simulink model "DriveTrain"  (R2019b)
settings: Solver=VariableStepAuto  StartTime=0.0  StopTime=30  RelTol=1e-3
settings Model: Creator=jorge  LastModifiedBy=jorge

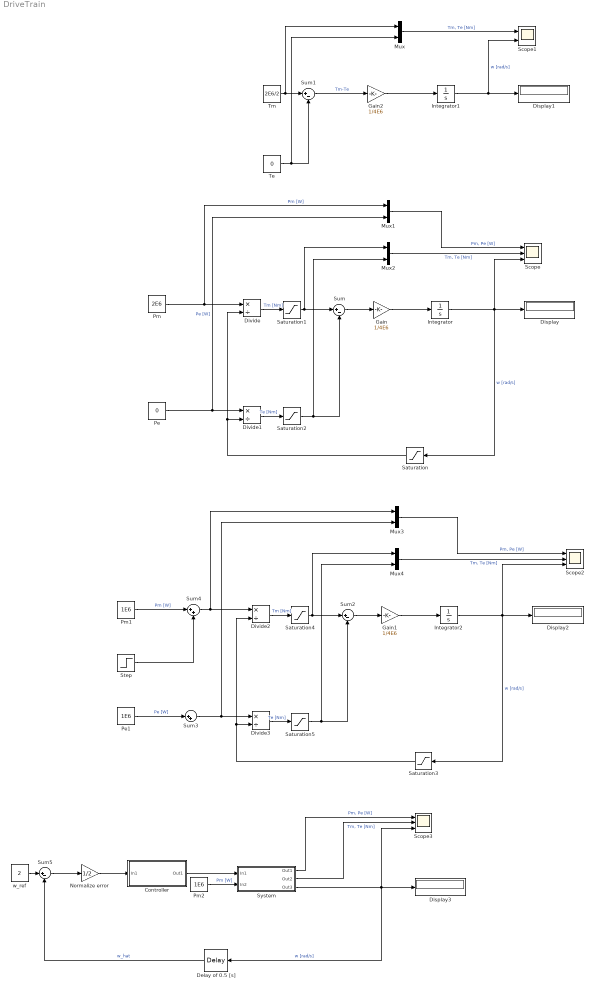
== system DriveTrain ==
  Controller : Subsystem
  Delay of 0.5 [s] : TransportDelay  DelayTime=0.5
  Display{,1..3} (4 alike) : Display
  Divide{,1..3} (4 alike) : Product  Inputs=*/
  Gain : Gain  Gain=1/4E6
  Gain1 : Gain  Gain=1/4E6
  Gain2 : Gain  Gain=1/4E6
  Integrator : Integrator
  Integrator1 : Integrator
  Integrator2 : Integrator  InitialCondition=2
  Mux{,1..4} (5 alike) : Mux  Inputs=2
  Normalize error : Gain  Gain=1/2
  Pe : Constant  Value=0
  Pe1 : Constant  Value=1E6
  Pm : Constant  Value=2E6
  Pm1 : Constant  Value=1E6
  Pm2 : Constant  Value=1E6
  Saturation : Saturate  UpperLimit=inf  LowerLimit=0.001
  Saturation1 : Saturate  UpperLimit=2E6
  Saturation2 : Saturate  UpperLimit=2E6  LowerLimit=0
  Saturation3 : Saturate  UpperLimit=inf  LowerLimit=0.001
  Saturation4 : Saturate  UpperLimit=2E6
  Saturation5 : Saturate  UpperLimit=2E6  LowerLimit=0
  Scope : Scope  NumInputPorts=3
  Scope1 : Scope  NumInputPorts=2
  Scope2 : Scope  NumInputPorts=3
  Scope3 : Scope  NumInputPorts=3
  Step : Step  After=2E5  SampleTime=0
  Sum{,1..2,5} (4 alike) : Sum  Inputs=|+-
  Sum3 : Sum  Inputs=|++
  Sum4 : Sum  Inputs=|++
  System : Subsystem
  Te : Constant  Value=0
  Tm : Constant  Value=2E6/2
  w_ref : Constant  Value=2
  wires:
  Integrator/1 -> Scope/3, Saturation/1, Display/1  "w [rad/s]"
  Gain/1 -> Integrator/1
  Gain2/1 -> Integrator1/1
  Sum1/1 -> Gain2/1  "Tm-Te"
  Integrator1/1 -> Scope1/2, Display1/1  "w [rad/s]"
  Te/1 -> Mux/2, Sum1/2
  Tm/1 -> Mux/1, Sum1/1
  Pm/1 -> Mux1/1, Divide/1  "Pm [W]"
  Saturation/1 -> Divide1/2, Divide/2
  Mux/1 -> Scope1/1  "Tm, Te [Nm]"
  Pe/1 -> Mux1/2, Divide1/1  "Pe [W]"
  Mux1/1 -> Scope/1  "Pm, Pe [W]"
  Sum/1 -> Gain/1
  Mux2/1 -> Scope/2  "Tm, Te [Nm]"
  Saturation1/1 -> Mux2/1, Sum/1
  Divide/1 -> Saturation1/1  "Tm [Nm]"
  Divide1/1 -> Saturation2/1  "Te [Nm]"
  Saturation2/1 -> Mux2/2, Sum/2
  Saturation4/1 -> Mux4/1, Sum2/1
  Divide3/1 -> Saturation5/1  "Te [Nm]"
  Gain1/1 -> Integrator2/1
  Integrator2/1 -> Scope2/3, Saturation3/1, Display2/1  "w [rad/s]"
  Divide2/1 -> Saturation4/1  "Tm [Nm]"
  Mux4/1 -> Scope2/2  "Tm, Te [Nm]"
  Mux3/1 -> Scope2/1  "Pm, Pe [W]"
  Saturation5/1 -> Mux4/2, Sum2/2
  Sum2/1 -> Gain1/1
  Saturation3/1 -> Divide3/2, Divide2/2
  Sum3/1 -> Mux3/2, Divide3/1
  Pe1/1 -> Sum3/1  "Pe [W]"
  Sum4/1 -> Mux3/1, Divide2/1
  Pm1/1 -> Sum4/1  "Pm [W]"
  Step/1 -> Sum4/2
  Pm2/1 -> System/2(In2)  "Pm [W]"
  Controller/1(Out1) -> System/1(In1)
  w_ref/1 -> Sum5/1
  Delay of 0.5 [s]/1 -> Sum5/2  "w_hat"
  System/1(Out1) -> Scope3/1  "Pm, Pe [W]"
  System/2(Out2) -> Scope3/2  "Tm, Te [Nm]"
  System/3(Out3) -> Scope3/3, Delay of 0.5 [s]/1, Display3/1  "w [rad/s]"
  Sum5/1 -> Normalize error/1
  Normalize error/1 -> Controller/1(In1)

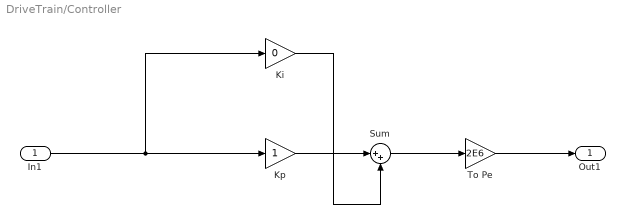
== system DriveTrain/Controller ==
  In1 : Inport
  Ki : Gain  Gain=0
  Kp : Gain
  Sum : Sum  Inputs=|++
  To Pe : Gain  Gain=2E6
  Out1 : Outport
  wires:
  In1/1 -> Ki/1, Kp/1
  Ki/1 -> Sum/2
  Kp/1 -> Sum/1
  Sum/1 -> To Pe/1
  To Pe/1 -> Out1/1

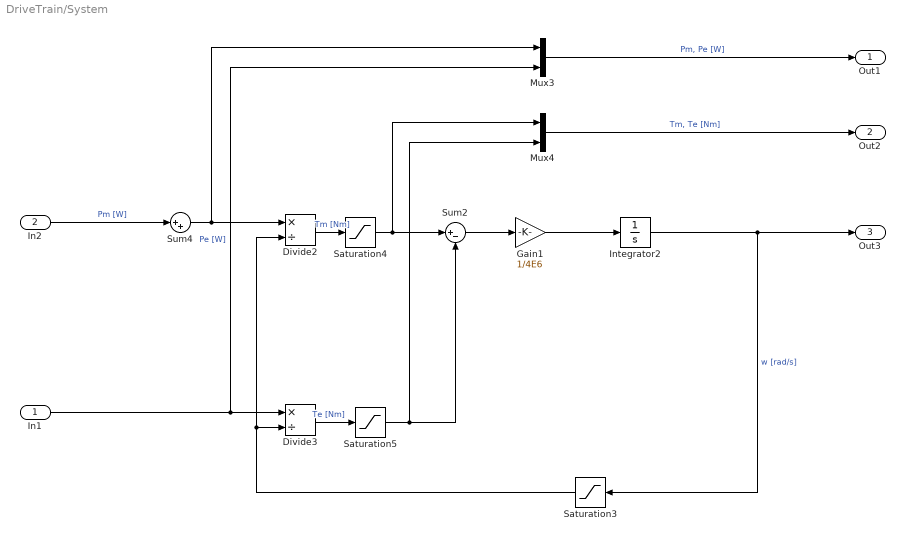
== system DriveTrain/System ==
  In1 : Inport
  In2 : Inport  Port=2
  Divide2 : Product  Inputs=*/
  Divide3 : Product  Inputs=*/
  Gain1 : Gain  Gain=1/4E6
  Integrator2 : Integrator  InitialCondition=2
  Mux3 : Mux  Inputs=2
  Mux4 : Mux  Inputs=2
  Saturation3 : Saturate  UpperLimit=inf  LowerLimit=0.001
  Saturation4 : Saturate  UpperLimit=2E6
  Saturation5 : Saturate  UpperLimit=2E6  LowerLimit=0
  Sum2 : Sum  Inputs=|+-
  Sum4 : Sum  Inputs=|++
  Out1 : Outport
  Out2 : Outport  Port=2
  Out3 : Outport  Port=3
  wires:
  In2/1 -> Sum4/1  "Pm [W]"
  Saturation3/1 -> Divide3/2, Divide2/2
  Sum2/1 -> Gain1/1
  Saturation5/1 -> Mux4/2, Sum2/2
  Mux4/1 -> Out2/1  "Tm, Te [Nm]"
  Mux3/1 -> Out1/1  "Pm, Pe [W]"
  Gain1/1 -> Integrator2/1
  Integrator2/1 -> Saturation3/1, Out3/1  "w [rad/s]"
  Divide3/1 -> Saturation5/1  "Te [Nm]"
  Saturation4/1 -> Mux4/1, Sum2/1
  Sum4/1 -> Mux3/1, Divide2/1
  Divide2/1 -> Saturation4/1  "Tm [Nm]"
  In1/1 -> Mux3/2, Divide3/1  "Pe [W]"
